simulink model "HelicPlantMRAC"  (Simulink 10.2)
settings: Solver=ode45  StartTime=0.0  StopTime=50.0  RelTol=1e-3  EnableMultiTasking=on
values from neighbouring files (symbols this model uses):
  am = -4    [init_mrac.m]    (also in init_mraclb.m = [0 1; -wn^2 -2*zet*wn])
  bb0 = -1    [init_mrac.m]
  bm = 4    [init_mrac.m]    (also in init_mraclb.m = [0; wn^2])
  gphi = 0.1    [init_mrac.m]
  gr = 0.0005    [init_mrac.m]
  gx = 0.0005    [init_mrac.m]
  k0 = 0    [init_mrac.m]
  ke = 10    [init_mrac.m]
  l0 = 0    [init_mrac.m]
  p = -1/(2*am)    (= 0.125)    [init_mrac.m]
  R = 0.15    [init_mrac.m]    (also in init_mraclb.m = 1.5)
  sigma2e = 0.01    [init_miac.m]    (also in init_mrac.m = 0; init_mraclb.m = 0)
  Tc = 0.1    [init_adrc.m]    (also in init_miac.m = 0.001; init_mrac.m; init_mraclb.m)
  theta0 = 0    [init_mrac.m]
  wr = 0.25    [init_miac.m]    (also in init_mrac.m; init_mraclb.m = 0.15)
libraries: simulink x1
settings Model: Creator=Melkamu A  LastModifiedBy=Melkamu A
settings DataIOCC: LimitDataPoints=on
settings OptimizationCC: InitFltsAndDblsToZero=on
settings DebuggingCC: SaveWithParameterizedLinksMsg=none  SignalResolutionControl=TryResolveAllWithWarning  SolverPrmCheckMsg=warning  MultiTaskDSMMsg=warning  MultiTaskCondExecSysMsg=none
settings SFSimCC: SimUseLocalCustomCode=on  CustomCodeUndefinedFunction=FilterOut
settings RTWCC: RTWUseLocalCustomCode=on
settings GRTTargetCC: TargetFcnLib=ansi_tfl_tmw.mat
settings ConfigComp: CovExternalEMLEnable=on

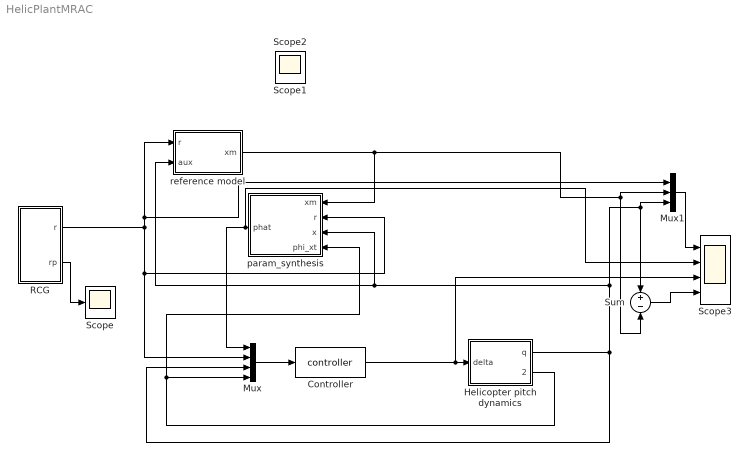
== system HelicPlantMRAC ==
  Controller : MATLABFcn  MATLABFcn=controller  OutputDimensions=1
  Helicopter pitch dynamics : Subsystem
  Mux : Mux  Inputs=[3 1 1 1]
  Mux1 : Mux  Inputs=3
  RCG : Subsystem
  Scope : Scope
  Scope3 : Scope  NumInputPorts=4
  Sum : Sum  Inputs=+-
  param_synthesis : Subsystem
  reference model : Subsystem
  Scope1 : Scope
  Scope2 : Scope
  wires:
  Helicopter pitch dynamics/1(q) -> Sum/1, Mux1/3, reference model/2(aux), param_synthesis/3(x), Mux/3
  RCG/1(r) -> Mux1/1, reference model/1(r), Mux/2, param_synthesis/2(r)
  Mux/1 -> Controller/1
  reference model/1(xm) -> param_synthesis/1(xm), Sum/2, Mux1/2
  param_synthesis/1(phat) -> Scope3/2, Mux/1
  Controller/1 -> Scope3/3, Helicopter pitch dynamics/1(delta)
  Helicopter pitch dynamics/2(phi_xt) -> Mux/4, param_synthesis/4(phi_xt)
  Sum/1 -> Scope3/4
  Mux1/1 -> Scope3/1
  RCG/2(rp) -> Scope/1

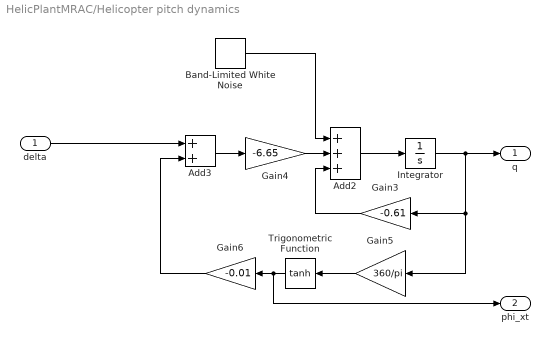
== system HelicPlantMRAC/Helicopter pitch dynamics ==
  delta : Inport
  Add2 : Sum  Inputs=+++
  Add3 : Sum
  Band-Limited White Noise : simulink/Sources/Band-Limited White Noise  Cov=[sigma2e*Tc]  Ts=Tc  seed=[23341]
  Gain3 : Gain  Gain=-0.61
  Gain4 : Gain  Gain=-6.65
  Gain5 : Gain  Gain=360/pi
  Gain6 : Gain  Gain=-0.01
  Integrator : Integrator  UpperSaturationLimit=100  LowerSaturationLimit=-100
  Trigonometric Function : Trigonometry  Operator=tanh
  q : Outport
  phi_xt : Outport  Port=2
  wires:
  Integrator/1 -> Gain3/1, Gain5/1, q/1
  Add2/1 -> Integrator/1
  Gain5/1 -> Trigonometric Function/1
  Trigonometric Function/1 -> phi_xt/1, Gain6/1
  Add3/1 -> Gain4/1
  Gain6/1 -> Add3/2
  delta/1 -> Add3/1
  Gain3/1 -> Add2/3
  Gain4/1 -> Add2/2
  Band-Limited White Noise/1 -> Add2/1

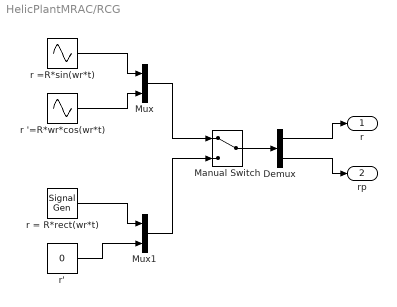
== system HelicPlantMRAC/RCG ==
  Demux : Demux  Outputs=2
  Manual Switch : ManualSwitch
  Mux : Mux  Inputs=2
  Mux1 : Mux  Inputs=2
  r '=R*wr*cos(wr*t) : Sin  Amplitude=R*wr  Frequency=wr  Phase=pi/2  SampleTime=0
  r = R*rect(wr*t) : SignalGenerator  WaveForm=square  Amplitude=R  Frequency=0.25  Units=rad/sec
  r =R*sin(wr*t) : Sin  Amplitude=R  Frequency=wr  SampleTime=0
  r' : Constant  Value=0
  r : Outport
  rp : Outport  Port=2
  wires:
  r =R*sin(wr*t)/1 -> Mux/1
  r '=R*wr*cos(wr*t)/1 -> Mux/2
  r = R*rect(wr*t)/1 -> Mux1/1
  r'/1 -> Mux1/2
  Mux/1 -> Manual Switch/1
  Mux1/1 -> Manual Switch/2
  Manual Switch/1 -> Demux/1
  Demux/1 -> r/1
  Demux/2 -> rp/1

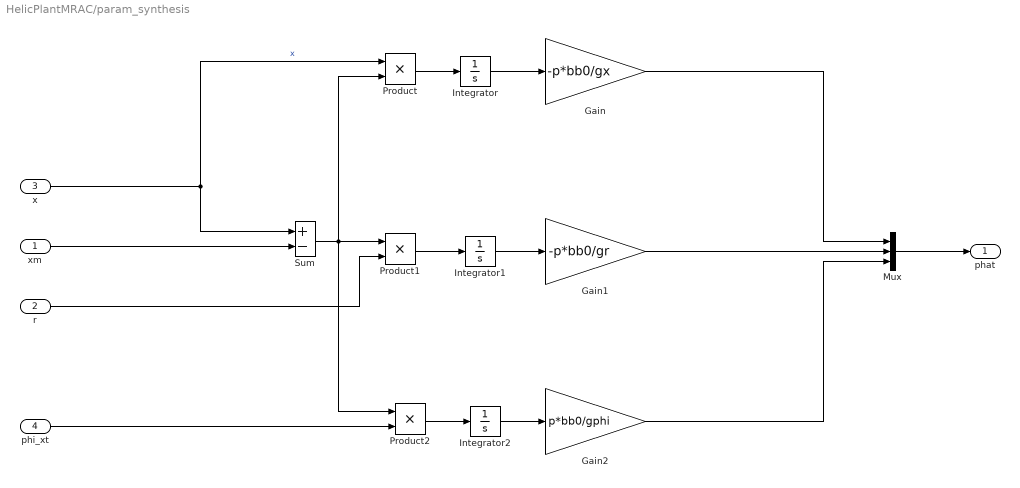
== system HelicPlantMRAC/param_synthesis ==
  xm : Inport
  r : Inport  Port=2
  x : Inport  Port=3
  phi_xt : Inport  Port=4
  Gain : Gain  Gain=-p*bb0/gx
  Gain1 : Gain  Gain=-p*bb0/gr
  Gain2 : Gain  Gain=p*bb0/gphi
  Integrator : Integrator  InitialCondition=k0
  Integrator1 : Integrator  InitialCondition=l0
  Integrator2 : Integrator  InitialCondition=theta0
  Mux : Mux  Inputs=3
  Product : Product
  Product1 : Product
  Product2 : Product
  Sum : Sum  Inputs=+-
  phat : Outport
  wires:
  Sum/1 -> Product/2, Product2/1, Product1/1
  x/1 -> Sum/1, Product/1  "x"
  Product/1 -> Integrator/1
  r/1 -> Product1/2
  Product1/1 -> Integrator1/1
  Product2/1 -> Integrator2/1
  phi_xt/1 -> Product2/2
  Mux/1 -> phat/1
  xm/1 -> Sum/2
  Gain1/1 -> Mux/2
  Gain/1 -> Mux/1
  Gain2/1 -> Mux/3
  Integrator2/1 -> Gain2/1
  Integrator1/1 -> Gain1/1
  Integrator/1 -> Gain/1

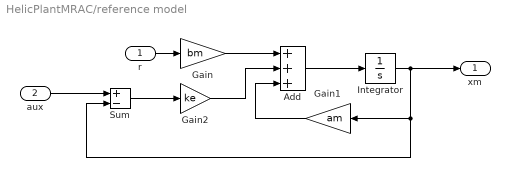
== system HelicPlantMRAC/reference model ==
  r : Inport
  aux : Inport  Port=2
  Add : Sum  Inputs=+++
  Gain : Gain  Gain=bm
  Gain1 : Gain  Gain=am
  Gain2 : Gain  Gain=ke
  Integrator : Integrator
  Sum : Sum  Inputs=+-
  xm : Outport
  wires:
  Gain/1 -> Add/1
  Add/1 -> Integrator/1
  Integrator/1 -> Sum/2, Gain1/1, xm/1
  r/1 -> Gain/1
  Gain1/1 -> Add/3
  aux/1 -> Sum/1
  Gain2/1 -> Add/2
  Sum/1 -> Gain2/1
